simulink model "inner_pd_test"  (R2015b)
settings: Solver=VariableStepAuto  StartTime=0.0  StopTime=50  RelTol=1e-3
undefined symbols (not defined in the file or in its folder): innerLoopSampleRate, omegalim, seed
settings Model: Creator=Daniel  LastModifiedBy=mgreiff

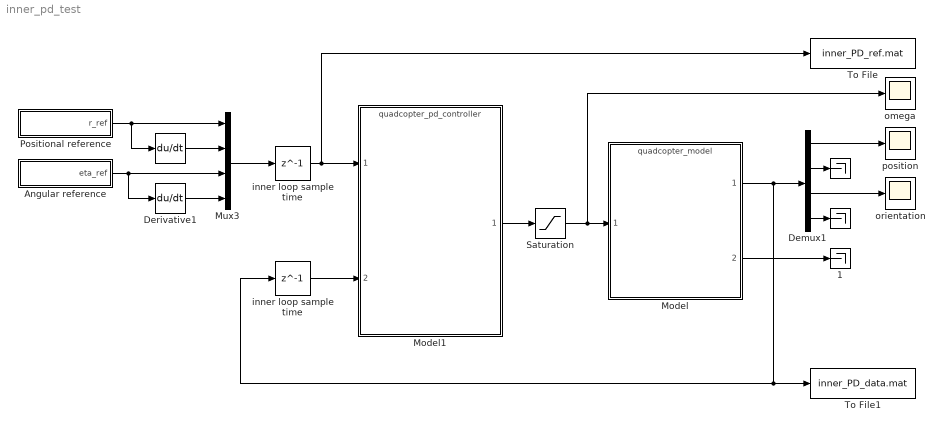
== system inner_pd_test ==
  "  " : Terminator
  "   " : Terminator
  "        " : Derivative
  "   1" : Terminator
  Angular reference : Subsystem
  Demux1 : Demux  Outputs=[3,3,3,3]
  Derivative1 : Derivative
  Model : ModelReference  ModelNameDialog=quadcopter_model.mdl  SimulationMode=Normal  ModelReferenceVersion=1.117  CopyOfModelName=quadcopter_model.mdl
  Model1 : ModelReference  ModelNameDialog=quadcopter_pd_controller.mdl  SimulationMode=Normal  ModelReferenceVersion=1.68  CopyOfModelName=quadcopter_pd_controller.mdl
  Mux3 : Mux  Inputs=[3,3,3,3]
  Positional reference : Subsystem
  Saturation : Saturate  UpperLimit=omegalim(2)  LowerLimit=omegalim(1)
  To File : ToFile  Filename=inner_PD_ref.mat  MatrixName=PD_ref  SaveFormat=Timeseries  SampleTime=innerLoopSampleRate
  To File1 : ToFile  Filename=inner_PD_data.mat  MatrixName=PD_data  SaveFormat=Timeseries  SampleTime=innerLoopSampleRate
  inner loop sample time : Delay  DelayLength=1  InitialCondition=0  SampleTime=innerLoopSampleRate
  "inner loop sample time " : Delay  DelayLength=1  InitialCondition=0  SampleTime=innerLoopSampleRate
  "omega " : Scope
  orientation : Scope
  position : Scope
  wires:
  Model1/1 -> Saturation/1
  Saturation/1 -> Model/1, "omega "/1
  Model/2 -> "   1"/1
  Demux1/2 -> "  "/1
  Demux1/4 -> "   "/1
  Demux1/1 -> position/1
  Demux1/3 -> orientation/1
  Angular reference/1(eta_ref) -> Derivative1/1, Mux3/3
  Positional reference/1(r_ref) -> Mux3/1, "        "/1
  "        "/1 -> Mux3/2
  Derivative1/1 -> Mux3/4
  Model/1 -> inner loop sample time/1, To File1/1, Demux1/1
  Mux3/1 -> "inner loop sample time "/1
  inner loop sample time/1 -> Model1/2
  "inner loop sample time "/1 -> Model1/1, To File/1

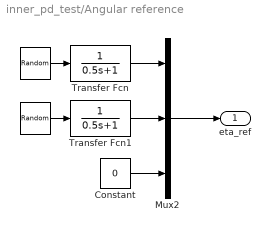
== system inner_pd_test/Angular reference ==
  " " : UniformRandomNumber  Minimum=-0.2  Maximum=0.2  Seed=4+seed  SampleTime=10
  "   " : UniformRandomNumber  Minimum=-0.2  Maximum=0.2  Seed=3+seed  SampleTime=10
  Constant : Constant  Value=0
  Mux2 : Mux  Inputs=3
  Transfer Fcn : TransferFcn  Denominator=[0.5 1]
  Transfer Fcn1 : TransferFcn  Denominator=[0.5 1]
  eta_ref : Outport
  wires:
  Mux2/1 -> eta_ref/1
  "   "/1 -> Transfer Fcn/1
  " "/1 -> Transfer Fcn1/1
  Transfer Fcn/1 -> Mux2/1
  Transfer Fcn1/1 -> Mux2/2
  Constant/1 -> Mux2/3

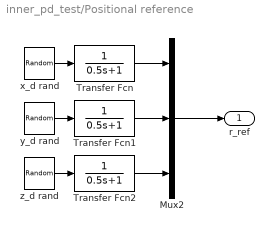
== system inner_pd_test/Positional reference ==
  Mux2 : Mux  Inputs=3
  Transfer Fcn : TransferFcn  Denominator=[0.5 1]
  Transfer Fcn1 : TransferFcn  Denominator=[0.5 1]
  Transfer Fcn2 : TransferFcn  Denominator=[0.5 1]
  x_d rand : UniformRandomNumber  Minimum=-30  Maximum=30  Seed=0+seed  SampleTime=10
  y_d rand : UniformRandomNumber  Minimum=-30  Maximum=30  Seed=1+seed  SampleTime=10
  z_d rand : UniformRandomNumber  Minimum=0  Maximum=15  Seed=2+seed  SampleTime=10
  r_ref : Outport
  wires:
  Mux2/1 -> r_ref/1
  x_d rand/1 -> Transfer Fcn/1
  y_d rand/1 -> Transfer Fcn1/1
  z_d rand/1 -> Transfer Fcn2/1
  Transfer Fcn/1 -> Mux2/1
  Transfer Fcn1/1 -> Mux2/2
  Transfer Fcn2/1 -> Mux2/3
